simulink model "multicoptero"  (R2021b)
settings: Solver=FixedStepAuto  StartTime=0.0  StopTime=10  FixedStep=1e-3  RelTol=1e-3
values from neighbouring files (symbols this model uses):
  controlador = projetarControladorArfagem(requisitos, planta)    [avaliarMalhaArfagem.m]    (also in avaliarMalhaVerticalPreFiltro.m = projetarControladorVerticalAnalitico(requisitos, planta); fazerTodosExperimentos.m = projetarControladorMulticoptero(req, planta); projetarControladorHorizontalBusca.m = projetarControladorHorizontalAnalitico(requisitoX, planta); projetarControladorVerticalBusca.m = projetarControladorVerticalAnalitico(requisito, planta))
  planta = obterPlantaMulticoptero()    [avaliarMalhaArfagem.m]    (also in avaliarMalhaHorizontal.m; avaliarMalhaVertical.m; avaliarMalhaVerticalPreFiltro.m; fazerTodosExperimentos.m)
undefined symbols (not defined in the file or in its folder): carga, theta0, ventoX
libraries: slpidlib x2
settings Model: Creator=mmaximo  LastModifiedBy=Eric
settings SolverCC: AlgebraicLoopSolver=TrustRegion
settings DebuggingCC: SFMachineParentedDataDiag=warning

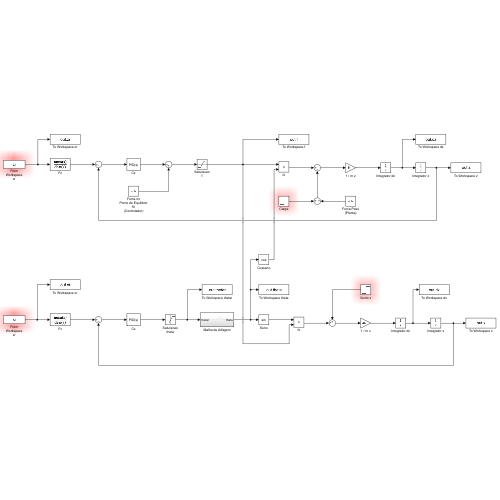
[thumbnail: Simulink's stored preview of the top-level diagram]
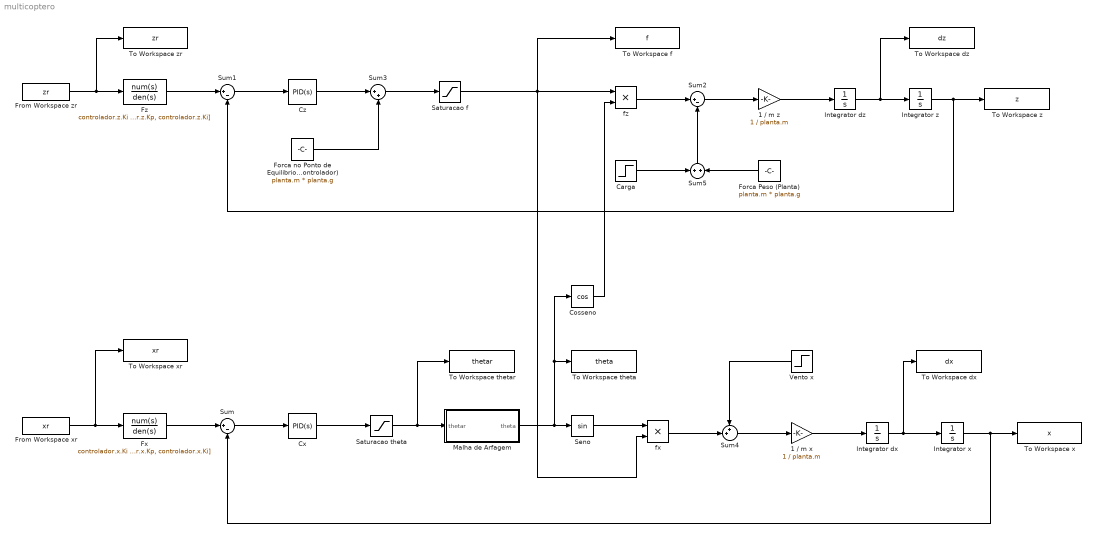
== system multicoptero ==
  1 / m x : Gain  Gain=1 / planta.m
  1 / m z : Gain  Gain=1 / planta.m
  Carga : Step  Time=3  After=carga * planta.g  SampleTime=0
  Cosseno : Trigonometry  Operator=cos
  Cx : slpidlib/PID Controller  Controller=PID  Form=Parallel  TimeDomain=Continuous-time  UseExternalTs=off  SampleTime=-1  IntegratorMethod=Forward Euler  FilterMethod=Forward Euler  ControllerParametersSource=internal  P=controlador.x.Kp  I=controlador.x.Ki  D=controlador.x.Kd  UseFilter=on  N=100  TunerSelectOption=Transfer Function Based (PID Tuner App)  InitialConditionSource=internal  InitialConditionForIntegrator=0  InitialConditionForFilter=0  DifferentiatorICPrevScaledInput=0  ExternalReset=none  TrackingMode=off  Kt=1  LimitOutput=off  SatLimitsSource=internal  UpperSaturationLimit=inf  LowerSaturationLimit=-inf  LinearizeAsGain=on  AntiWindupMode=none  Kb=1  POutMin=[]  POutMax=[]  IOutMin=[]  IOutMax=[]  DOutMin=[]  DOutMax=[]  NOutMin=[]  NOutMax=[]  SumOutMin=[]  SumOutMax=[]  SaturationOutMin=[]  SaturationOutMax=[]  PParamMin=[]  PParamMax=[]  IParamMin=[]  IParamMax=[]  DParamMin=[]  DParamMax=[]  NParamMin=[]  NParamMax=[]  KbParamMin=[]  KbParamMax=[]  KtParamMin=[]  KtParamMax=[]  KbOutMin=[]  KbOutMax=[]  KtOutMin=[]  KtOutMax=[]  IntegratorOutMin=[]  IntegratorOutMax=[]  FilterOutMin=[]  FilterOutMax=[]  SumI1OutMin=[]  SumI1OutMax=[]  SumI2OutMin=[]  SumI2OutMax=[]  SumI3OutMin=[]  SumI3OutMax=[]  SumI4OutMin=[]  SumI4OutMax=[]  SumDOutMin=[]  SumDOutMax=[]  DifferentiatorOutMin=[]  DifferentiatorOutMax=[]  FilterDiffOutCoefMin=[]  FilterDiffOutCoefMax=[]  ReciprocalOutMin=[]  ReciprocalOutMax=[]  SumDenOutMin=[]  SumDenOutMax=[]  SumNumOutMin=[]  SumNumOutMax=[]  DivideOutMin=[]  DivideOutMax=[]  UdiffTsProdOutMin=[]  UdiffTsProdOutMax=[]  NTsProdOutMin=[]  NTsProdOutMax=[]  UintegralTsProdOutMin=[]  UintegralTsProdOutMax=[]  UngainTsProdOutMin=[]  UngainTsProdOutMax=[]  IntegratorContinuousStateAttributes=''  IntegratorStateMustResolveToSignalObject=off  IntegratorRTWStateStorageClass=Auto  FilterContinuousStateAttributes=''  FilterStateMustResolveToSignalObject=off  FilterRTWStateStorageClass=Auto  ParallelPVariant=InternalParameters  IdealPVariant=Disabled  IVariant=InternalParameters  DVariant=InternalParameters  IntegratorVariant=Continuous  SatVariant=Disabled  AWVariant=Passthrough  PCopyVariant=Disabled  TRVariant=Disabled  FdbkBlocksVariant=Forward  IdealPFdbkVariant=Disabled  SatFdbkVariant=Disabled  DerivativeFilterVariant=ContFilter  NVariant=InternalParameters  NCopyVariant=Disabled  FilterICVariant=InternalICsFilter  IntegratorICVariant=InternalICs  ExternalResetVariant=Disabled  TRSumVariant=Passthrough  SumFdbkVariant=Disabled  SumVariant=Sum_PID  TsampFilterVariant=InternalTs  TsampNgainVariant=Passthrough  TsampIntegralVariant=Passthrough  ExternalSaturationOutDataTypeStr=Inherit: Same as second input
  Cz : slpidlib/PID Controller  Controller=PID  Form=Parallel  TimeDomain=Continuous-time  UseExternalTs=off  SampleTime=-1  IntegratorMethod=Forward Euler  FilterMethod=Forward Euler  ControllerParametersSource=internal  P=controlador.z.Kp  I=controlador.z.Ki  D=controlador.z.Kd  UseFilter=on  N=100  TunerSelectOption=Transfer Function Based (PID Tuner App)  InitialConditionSource=internal  InitialConditionForIntegrator=0  InitialConditionForFilter=0  DifferentiatorICPrevScaledInput=0  ExternalReset=none  TrackingMode=off  Kt=1  LimitOutput=off  SatLimitsSource=internal  UpperSaturationLimit=inf  LowerSaturationLimit=-inf  LinearizeAsGain=on  AntiWindupMode=none  Kb=1  POutMin=[]  POutMax=[]  IOutMin=[]  IOutMax=[]  DOutMin=[]  DOutMax=[]  NOutMin=[]  NOutMax=[]  SumOutMin=[]  SumOutMax=[]  SaturationOutMin=[]  SaturationOutMax=[]  PParamMin=[]  PParamMax=[]  IParamMin=[]  IParamMax=[]  DParamMin=[]  DParamMax=[]  NParamMin=[]  NParamMax=[]  KbParamMin=[]  KbParamMax=[]  KtParamMin=[]  KtParamMax=[]  KbOutMin=[]  KbOutMax=[]  KtOutMin=[]  KtOutMax=[]  IntegratorOutMin=[]  IntegratorOutMax=[]  FilterOutMin=[]  FilterOutMax=[]  SumI1OutMin=[]  SumI1OutMax=[]  SumI2OutMin=[]  SumI2OutMax=[]  SumI3OutMin=[]  SumI3OutMax=[]  SumI4OutMin=[]  SumI4OutMax=[]  SumDOutMin=[]  SumDOutMax=[]  DifferentiatorOutMin=[]  DifferentiatorOutMax=[]  FilterDiffOutCoefMin=[]  FilterDiffOutCoefMax=[]  ReciprocalOutMin=[]  ReciprocalOutMax=[]  SumDenOutMin=[]  SumDenOutMax=[]  SumNumOutMin=[]  SumNumOutMax=[]  DivideOutMin=[]  DivideOutMax=[]  UdiffTsProdOutMin=[]  UdiffTsProdOutMax=[]  NTsProdOutMin=[]  NTsProdOutMax=[]  UintegralTsProdOutMin=[]  UintegralTsProdOutMax=[]  UngainTsProdOutMin=[]  UngainTsProdOutMax=[]  IntegratorContinuousStateAttributes=''  IntegratorStateMustResolveToSignalObject=off  IntegratorRTWStateStorageClass=Auto  FilterContinuousStateAttributes=''  FilterStateMustResolveToSignalObject=off  FilterRTWStateStorageClass=Auto  ParallelPVariant=InternalParameters  IdealPVariant=Disabled  IVariant=InternalParameters  DVariant=InternalParameters  IntegratorVariant=Continuous  SatVariant=Disabled  AWVariant=Passthrough  PCopyVariant=Disabled  TRVariant=Disabled  FdbkBlocksVariant=Forward  IdealPFdbkVariant=Disabled  SatFdbkVariant=Disabled  DerivativeFilterVariant=ContFilter  NVariant=InternalParameters  NCopyVariant=Disabled  FilterICVariant=InternalICsFilter  IntegratorICVariant=InternalICs  ExternalResetVariant=Disabled  TRSumVariant=Passthrough  SumFdbkVariant=Disabled  SumVariant=Sum_PID  TsampFilterVariant=InternalTs  TsampNgainVariant=Passthrough  TsampIntegralVariant=Passthrough  ExternalSaturationOutDataTypeStr=Inherit: Same as second input
  Forca Peso (Planta) : Constant  Value=planta.m * planta.g
  Forca no Ponto de Equilibrio f0 (Controlador) : Constant  Value=planta.m * planta.g
  From Workspace xr : FromWorkspace  VariableName=xr
  From Workspace zr : FromWorkspace  VariableName=zr
  Fx : TransferFcn  Numerator=controlador.x.Ki  Denominator=[controlador.x.Kd, controlador.x.Kp, controlador.x.Ki]
  Fz : TransferFcn  Numerator=controlador.z.Ki  Denominator=[controlador.z.Kd, controlador.z.Kp, controlador.z.Ki]
  Integrator dx : Integrator
  Integrator dz : Integrator
  Integrator x : Integrator
  Integrator z : Integrator
  Malha de Arfagem : Subsystem
  Saturacao f : Saturate  UpperLimit=1.8 * planta.m * planta.g  LowerLimit=0.2 * planta.m * planta.g
  Saturacao theta : Saturate  UpperLimit=80 * pi / 180  LowerLimit=-80 * pi / 180
  Seno : Trigonometry
  Sum : Sum  Inputs=|+-
  Sum1 : Sum  Inputs=|+-
  Sum2 : Sum  Inputs=|+-
  Sum3 : Sum  Inputs=|++
  Sum4 : Sum  Inputs=++|
  Sum5 : Sum  Inputs=+|+
  To Workspace dx : ToWorkspace  VariableName=dx  SaveFormat=Structure With Time  SampleTime=-1
  To Workspace dz : ToWorkspace  VariableName=dz  SaveFormat=Structure With Time  SampleTime=-1
  To Workspace f : ToWorkspace  VariableName=f  SaveFormat=Structure With Time  SampleTime=-1
  To Workspace theta : ToWorkspace  VariableName=theta  SaveFormat=Structure With Time  SampleTime=-1
  To Workspace thetar : ToWorkspace  VariableName=thetar  SaveFormat=Structure With Time  SampleTime=-1
  To Workspace x : ToWorkspace  VariableName=x  SaveFormat=Structure With Time  SampleTime=-1
  To Workspace xr : ToWorkspace  VariableName=xr  SaveFormat=Structure With Time  SampleTime=-1
  To Workspace z : ToWorkspace  VariableName=z  SaveFormat=Structure With Time  SampleTime=-1
  To Workspace zr : ToWorkspace  VariableName=zr  SaveFormat=Structure With Time  SampleTime=-1
  Vento x : Step  Time=3  After=ventoX  SampleTime=0
  fx : Product
  fz : Product
  wires:
  Cosseno/1 -> fz/2
  Seno/1 -> fx/1
  Cz/1 -> Sum3/1
  Forca no Ponto de Equilibrio f0 (Controlador)/1 -> Sum3/2
  Integrator dx/1 -> To Workspace dx/1, Integrator x/1
  Integrator dz/1 -> Integrator z/1, To Workspace dz/1
  Integrator z/1 -> Sum1/2, To Workspace z/1
  Integrator x/1 -> Sum/2, To Workspace x/1
  From Workspace zr/1 -> Fz/1, To Workspace zr/1
  Vento x/1 -> Sum4/1
  Sum4/1 -> 1 / m x/1
  Forca Peso (Planta)/1 -> Sum5/2
  Carga/1 -> Sum5/1
  Sum5/1 -> Sum2/2
  Saturacao f/1 -> fx/2, fz/1, To Workspace f/1
  Malha de Arfagem/1(theta) -> Seno/1, Cosseno/1, To Workspace theta/1
  Saturacao theta/1 -> Malha de Arfagem/1(thetar), To Workspace thetar/1
  Sum2/1 -> 1 / m z/1
  From Workspace xr/1 -> Fx/1, To Workspace xr/1
  Fx/1 -> Sum/1
  Fz/1 -> Sum1/1
  Sum1/1 -> Cz/1
  fz/1 -> Sum2/1
  1 / m z/1 -> Integrator dz/1
  Sum3/1 -> Saturacao f/1
  Sum/1 -> Cx/1
  Cx/1 -> Saturacao theta/1
  fx/1 -> Sum4/2
  1 / m x/1 -> Integrator dx/1

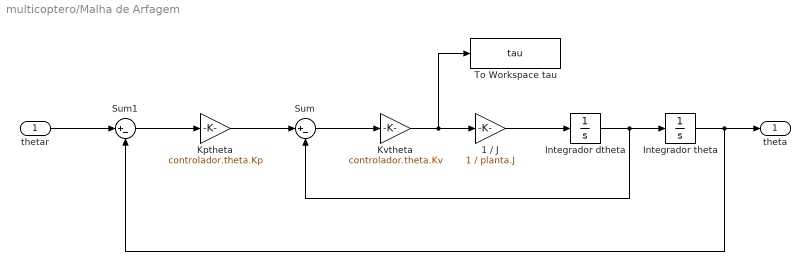
== system multicoptero/Malha de Arfagem ==
  thetar : Inport
  1 / J : Gain  Gain=1 / planta.J
  Integrador dtheta : Integrator
  Integrador theta : Integrator  InitialCondition=theta0
  Kptheta : Gain  Gain=controlador.theta.Kp
  Kvtheta : Gain  Gain=controlador.theta.Kv
  Sum : Sum  Inputs=|+-
  Sum1 : Sum  Inputs=|+-
  To Workspace tau : ToWorkspace  VariableName=tau  SaveFormat=Structure With Time  SampleTime=-1
  theta : Outport
  wires:
  Kvtheta/1 -> 1 / J/1, To Workspace tau/1
  thetar/1 -> Sum1/1
  Sum1/1 -> Kptheta/1
  Kptheta/1 -> Sum/1
  Sum/1 -> Kvtheta/1
  1 / J/1 -> Integrador dtheta/1
  Integrador dtheta/1 -> Sum/2, Integrador theta/1
  Integrador theta/1 -> Sum1/2, theta/1
